simulink model "sos_2"  (Simulink 6.1)
settings: Solver=ode45  StartTime=0.0  StopTime=10.0  RelTol=1e-3
libraries: dspsigops x4
settings Model: Creator=svenhoffmann  LastModifiedBy=svenhoffmann  ExtModeAutoUpdateStatusClock=off
settings DebuggingCC: SolverPrmCheckMsg=warning

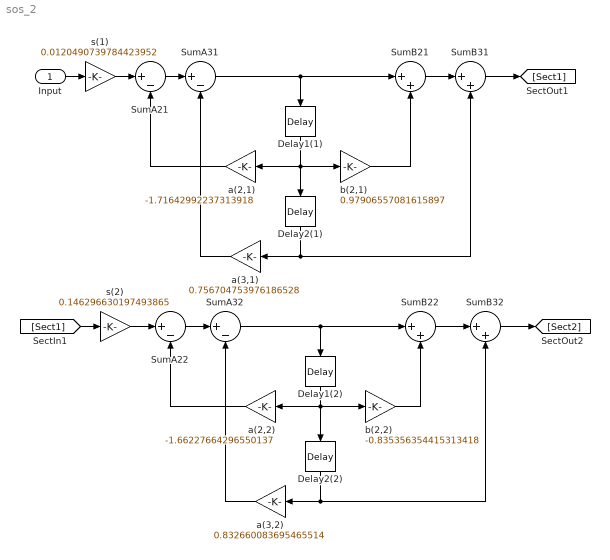
== system sos_2 ==
  Input : Inport  Port=1  LatchInput=off
  Delay1(1) : dspsigops/Delay  Orientation=down  dly_unit=Samples  delay=1  ic_detail=off  dif_ic_for_ch=off  dif_ic_for_dly=off  ic=0  reset_popup=None
  Delay1(2) : dspsigops/Delay  Orientation=down  dly_unit=Samples  delay=1  ic_detail=off  dif_ic_for_ch=off  dif_ic_for_dly=off  ic=0  reset_popup=None
  Delay2(1) : dspsigops/Delay  Orientation=down  dly_unit=Samples  delay=1  ic_detail=off  dif_ic_for_ch=off  dif_ic_for_dly=off  ic=0  reset_popup=None
  Delay2(2) : dspsigops/Delay  Orientation=down  dly_unit=Samples  delay=1  ic_detail=off  dif_ic_for_ch=off  dif_ic_for_dly=off  ic=0  reset_popup=None
  SumA{21..22,31..32} (4 alike) : Sum  Inputs=|+-  SaturateOnIntegerOverflow=on  InputSameDT=on
  SumB{21..22,31..32} (4 alike) : Sum  Inputs=|++  SaturateOnIntegerOverflow=on  InputSameDT=on
  a(2,1) : Gain  Orientation=left  Gain=-1.71642992237313918  SaturateOnIntegerOverflow=on
  a(2,2) : Gain  Orientation=left  Gain=-1.66227664296550137  SaturateOnIntegerOverflow=on
  a(3,1) : Gain  Orientation=left  Gain=0.756704753976186528  SaturateOnIntegerOverflow=on
  a(3,2) : Gain  Orientation=left  Gain=0.832660083695465514  SaturateOnIntegerOverflow=on
  b(2,1) : Gain  Gain=0.97906557081615897  SaturateOnIntegerOverflow=on
  b(2,2) : Gain  Gain=-0.835356354415313418  SaturateOnIntegerOverflow=on
  s(1) : Gain  Gain=0.0120490739784423952  SaturateOnIntegerOverflow=on
  s(2) : Gain  Gain=0.146296630197493865  SaturateOnIntegerOverflow=on
  wires:
  Input/1 -> s(1)/1
  s(1)/1 -> SumA21/1
  SumA21/1 -> SumA31/1
  SumA31/1 -> SumB21/1, Delay1(1)/1
  SumB21/1 -> SumB31/1
  SumB31/1 -> [Sect1]
  Delay1(1)/1 -> a(2,1)/1, b(2,1)/1, Delay2(1)/1
  b(2,1)/1 -> SumB21/2
  Delay2(1)/1 -> SumB31/2, a(3,1)/1
  a(2,1)/1 -> SumA21/2
  a(3,1)/1 -> SumA31/2
  [Sect1] -> s(2)/1
  s(2)/1 -> SumA22/1
  SumA22/1 -> SumA32/1
  SumA32/1 -> SumB22/1, Delay1(2)/1
  SumB22/1 -> SumB32/1
  SumB32/1 -> [Sect2]
  Delay1(2)/1 -> a(2,2)/1, b(2,2)/1, Delay2(2)/1
  b(2,2)/1 -> SumB22/2
  Delay2(2)/1 -> SumB32/2, a(3,2)/1
  a(2,2)/1 -> SumA22/2
  a(3,2)/1 -> SumA32/2
